simulink model "power_wind_dfig"  (R2016a)
settings: Solver=ode23tb  StartTime=0.0  StopTime=100  FixedStep=1/60  MaxStep=1/60  RelTol=1e-4  AbsTol=1e-3
InitFcn:
  | xInitial = init_power_wind_dfig;
undefined symbols (not defined in the file): b0, D1, D11, Delta, F, find_system, Fnom, gcbh, H, ILd_init, ILq_init, Imax_grid_conv, Init, j, Kd, Ki_dc_reg, Ki_grid_side_cur_reg, Ki_power_reg, Ki_Q, Ki_rotor_side_cur_reg, Ki_volt_reg, Kp, Kp_dc_reg, Kp_grid_side_cur_reg, Kp_power_reg, Kp_Q, Kp_rotor_side_cur_reg, Kp_volt_reg, L_RL, Llr, Lls, p, Pnom, power_A, power_B, power_D, R_RL, Rr, Rs, speed_A, speed_B, speed_C, speed_D, sps_rtmsupport, Vcontrol, Vnom, Wind_On, wo
libraries: powerlib_meascontrol x29, powerlib x27, simulink_extras x5, re_lib x2
(part 5 of 5)

== system power_wind_dfig/Plant 2 MVA/Plant & Motor Protection/AC Voltage Protection/Voltage Measurement/magnitude2/Fourier1 ==
  signal : Inport
  Constant : Constant  Value=0
  Fcn : Fcn  Expr=u^2
  Fcn1 : Fcn  Expr=u^2
  Fcn2 : Fcn  Expr=sqrt(u)
  Fcn3 : Fcn  Expr=180/pi*atan2(u[2],u[1])
  Gain1 : Gain  Gain=k*f1  SaturateOnIntegerOverflow=on  OutDataTypeStr=Inherit: Same as input  ParamDataTypeStr=Inherit: Same as input
  Integ2 : Integrator  InitialConditionSource=external
  Mux : Mux  Inputs=2
  Product : Product  SaturateOnIntegerOverflow=on  InputSameDT=on  OutDataTypeStr=Inherit: Same as first input
  Product1 : Product  SaturateOnIntegerOverflow=on  InputSameDT=on  OutDataTypeStr=Inherit: Same as first input
  Sum : Sum  SaturateOnIntegerOverflow=on  InputSameDT=on  OutDataTypeStr=Inherit: Same as first input
  Sum1 : Sum  Inputs=+-  SaturateOnIntegerOverflow=on  InputSameDT=on  OutDataTypeStr=Inherit: Same as first input
  Sum2 : Sum  Inputs=+-  SaturateOnIntegerOverflow=on  InputSameDT=on  OutDataTypeStr=Inherit: Same as first input
  T : TransportDelay  DelayTime=1/f1  BufferSize=2048
  T1 : TransportDelay  DelayTime=1/f1  BufferSize=2048
  cos(nwt) : Sin  Frequency=2*pi*n*f1  Phase=pi/2  SampleTime=0
  integ1 : Integrator  InitialConditionSource=external
  sin(nwt) : Sin  Frequency=2*pi*n*f1  SampleTime=0
  magnitude : Outport  InitialOutput=0
  angle : Outport  Port=2  InitialOutput=0
  wires:
  Constant/1 -> integ1/2, Integ2/2
  Sum/1 -> Fcn2/1
  Fcn/1 -> Sum/1
  Fcn1/1 -> Sum/2
  Mux/1 -> Fcn3/1
  Fcn3/1 -> angle/1
  sin(nwt)/1 -> Product/1
  cos(nwt)/1 -> Product1/2
  Product/1 -> integ1/1
  Product1/1 -> Integ2/1
  T/1 -> Sum1/2
  T1/1 -> Sum2/2
  integ1/1 -> Sum1/1, T/1
  Integ2/1 -> T1/1, Sum2/1
  Sum2/1 -> Fcn1/1, Mux/2
  Sum1/1 -> Fcn/1, Mux/1
  signal/1 -> Gain1/1
  Gain1/1 -> Product/2, Product1/1
  Fcn2/1 -> magnitude/1

== system power_wind_dfig/Plant 2 MVA/Plant & Motor Protection/AC Voltage Protection/Voltage Measurement/magnitude2/Fourier2 ==
  signal : Inport
  Constant : Constant  Value=0
  Fcn : Fcn  Expr=u^2
  Fcn1 : Fcn  Expr=u^2
  Fcn2 : Fcn  Expr=sqrt(u)
  Fcn3 : Fcn  Expr=180/pi*atan2(u[2],u[1])
  Gain1 : Gain  Gain=k*f1  SaturateOnIntegerOverflow=on  OutDataTypeStr=Inherit: Same as input  ParamDataTypeStr=Inherit: Same as input
  Integ2 : Integrator  InitialConditionSource=external
  Mux : Mux  Inputs=2
  Product : Product  SaturateOnIntegerOverflow=on  InputSameDT=on  OutDataTypeStr=Inherit: Same as first input
  Product1 : Product  SaturateOnIntegerOverflow=on  InputSameDT=on  OutDataTypeStr=Inherit: Same as first input
  Sum : Sum  SaturateOnIntegerOverflow=on  InputSameDT=on  OutDataTypeStr=Inherit: Same as first input
  Sum1 : Sum  Inputs=+-  SaturateOnIntegerOverflow=on  InputSameDT=on  OutDataTypeStr=Inherit: Same as first input
  Sum2 : Sum  Inputs=+-  SaturateOnIntegerOverflow=on  InputSameDT=on  OutDataTypeStr=Inherit: Same as first input
  T : TransportDelay  DelayTime=1/f1  BufferSize=2048
  T1 : TransportDelay  DelayTime=1/f1  BufferSize=2048
  cos(nwt) : Sin  Frequency=2*pi*n*f1  Phase=pi/2  SampleTime=0
  integ1 : Integrator  InitialConditionSource=external
  sin(nwt) : Sin  Frequency=2*pi*n*f1  SampleTime=0
  magnitude : Outport  InitialOutput=0
  angle : Outport  Port=2  InitialOutput=0
  wires:
  Fcn2/1 -> magnitude/1
  Gain1/1 -> Product1/1, Product/2
  signal/1 -> Gain1/1
  Sum1/1 -> Mux/1, Fcn/1
  Sum2/1 -> Mux/2, Fcn1/1
  Integ2/1 -> Sum2/1, T1/1
  integ1/1 -> T/1, Sum1/1
  T1/1 -> Sum2/2
  T/1 -> Sum1/2
  Product1/1 -> Integ2/1
  Product/1 -> integ1/1
  cos(nwt)/1 -> Product1/2
  sin(nwt)/1 -> Product/1
  Fcn3/1 -> angle/1
  Mux/1 -> Fcn3/1
  Fcn1/1 -> Sum/2
  Fcn/1 -> Sum/1
  Sum/1 -> Fcn2/1
  Constant/1 -> Integ2/2, integ1/2

== system power_wind_dfig/Wind Turbine Doubly-Fed Induction Generator (Phasor Type)1/Generator & Converters/Control/wind_dfig_grid/Current regulator/Subsystem3 ==
  In1 : Inport
  Gain : Gain  Gain=Ki  SaturateOnIntegerOverflow=on  OutDataTypeStr=Inherit: Same as input  ParamDataTypeStr=Inherit: Same as input
  Gain1 : Gain  Gain=Kp  SaturateOnIntegerOverflow=on  OutDataTypeStr=Inherit: Same as input  ParamDataTypeStr=Inherit: Same as input
  Integrator : Integrator  InitialCondition=Init  LimitOutput=on  UpperSaturationLimit=Upper_Limit  LowerSaturationLimit=Lower_Limit
  Saturation : Saturate  UpperLimit=Upper_Limit  LowerLimit=Lower_Limit
  Sum7 : Sum  SaturateOnIntegerOverflow=on  InputSameDT=on  OutDataTypeStr=Inherit: Same as first input
  Out1 : Outport
  wires:
  Saturation/1 -> Out1/1
  Sum7/1 -> Saturation/1
  In1/1 -> Gain/1, Gain1/1
  Integrator/1 -> Sum7/2
  Gain1/1 -> Sum7/1
  Gain/1 -> Integrator/1

== system power_wind_dfig/Wind Turbine Doubly-Fed Induction Generator (Phasor Type)1/Generator & Converters/Control/wind_dfig_grid/DC bus voltage Regulator/Subsystem1 ==
  In1 : Inport
  Gain : Gain  Gain=Ki  SaturateOnIntegerOverflow=on  OutDataTypeStr=Inherit: Same as input  ParamDataTypeStr=Inherit: Same as input
  Gain1 : Gain  Gain=Kp  SaturateOnIntegerOverflow=on  OutDataTypeStr=Inherit: Same as input  ParamDataTypeStr=Inherit: Same as input
  Integrator : Integrator  InitialCondition=Init  LimitOutput=on  UpperSaturationLimit=Upper_Limit  LowerSaturationLimit=Lower_Limit
  Saturation : Saturate  UpperLimit=Upper_Limit  LowerLimit=Lower_Limit
  Sum7 : Sum  SaturateOnIntegerOverflow=on  InputSameDT=on  OutDataTypeStr=Inherit: Same as first input
  Out1 : Outport
  wires:
  Saturation/1 -> Out1/1
  Sum7/1 -> Saturation/1
  In1/1 -> Gain/1, Gain1/1
  Integrator/1 -> Sum7/2
  Gain1/1 -> Sum7/1
  Gain/1 -> Integrator/1

== system power_wind_dfig/Wind Turbine Doubly-Fed Induction Generator (Phasor Type)1/Generator & Converters/Control/wind_dfig_rotor/Current Regulator/Subsystem1 ==
  In1 : Inport
  Gain : Gain  Gain=Ki  SaturateOnIntegerOverflow=on  OutDataTypeStr=Inherit: Same as input  ParamDataTypeStr=Inherit: Same as input
  Gain1 : Gain  Gain=Kp  SaturateOnIntegerOverflow=on  OutDataTypeStr=Inherit: Same as input  ParamDataTypeStr=Inherit: Same as input
  Integrator : Integrator  InitialCondition=Init  LimitOutput=on  UpperSaturationLimit=Upper_Limit  LowerSaturationLimit=Lower_Limit
  Saturation : Saturate  UpperLimit=Upper_Limit  LowerLimit=Lower_Limit
  Sum7 : Sum  SaturateOnIntegerOverflow=on  InputSameDT=on  OutDataTypeStr=Inherit: Same as first input
  Out1 : Outport
  wires:
  Saturation/1 -> Out1/1
  Sum7/1 -> Saturation/1
  In1/1 -> Gain/1, Gain1/1
  Integrator/1 -> Sum7/2
  Gain1/1 -> Sum7/1
  Gain/1 -> Integrator/1

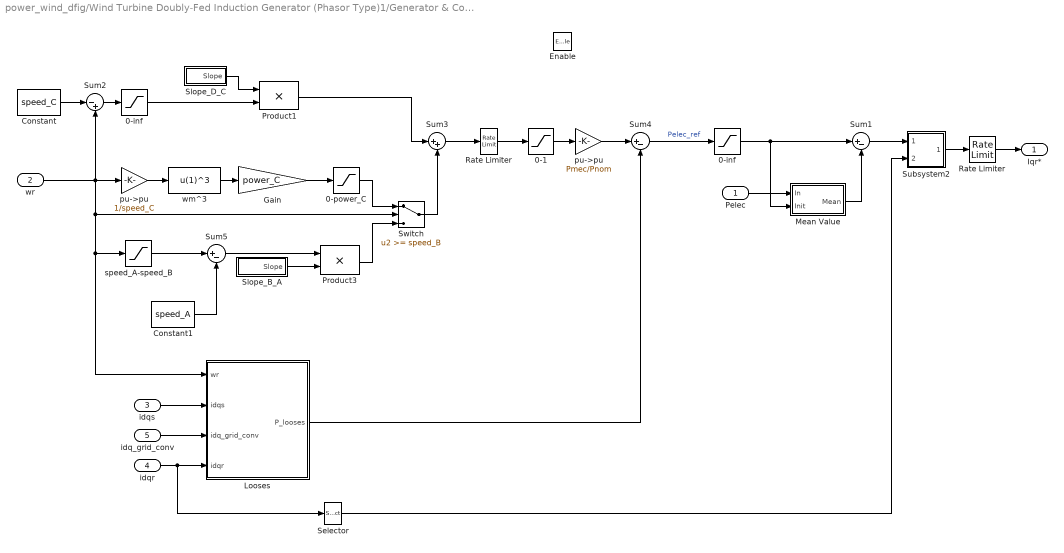
== system power_wind_dfig/Wind Turbine Doubly-Fed Induction Generator (Phasor Type)1/Generator & Converters/Control/wind_dfig_rotor/Power Regulator/Subsystem ==
  Pelec : Inport
  wr : Inport  Port=2
  idqs : Inport  Port=3
  idqr : Inport  Port=4
  idq_grid_conv : Inport  Port=5
  Enable : EnablePort  PropagateVarSize=During execution
  0-1 : Saturate  UpperLimit=1  LowerLimit=0
  0-inf : Saturate  UpperLimit=inf  LowerLimit=0
  "0-inf " : Saturate  UpperLimit=inf  LowerLimit=0
  0-power_C : Saturate  UpperLimit=power_C  LowerLimit=0
  Constant : Constant  Value=speed_C
  Constant1 : Constant  Value=speed_A
  "Gain " : Gain  Gain=power_C  SaturateOnIntegerOverflow=on  OutDataTypeStr=Inherit: Same as input  ParamDataTypeStr=Inherit: Same as input
  Looses : Subsystem
  Mean Value : Subsystem  mask(Mean value){Period=1/Fnom}
      mask prompts: Period "Averaging period (s):"
      mask help: This block uses the running window averaging technique to compute the mean value of the input signal over the specified period.
  Product1 : Product  SaturateOnIntegerOverflow=on  OutDataTypeStr=Inherit: Same as first input
  Product3 : Product  SaturateOnIntegerOverflow=on  OutDataTypeStr=Inherit: Same as first input
  Rate Limiter : RateLimiter  RisingSlewLimit=current_slew_rate  FallingSlewLimit=-current_slew_rate
  "Rate Limiter " : RateLimiter  RisingSlewLimit=power_slew_rate  FallingSlewLimit=-power_slew_rate
  Selector : Selector  InputPortWidth=2  IndexOptions=Index vector (dialog)  Indices=2  OutputSizes=1
  Slope_B_A : Subsystem
  Slope_D_C : Subsystem
  Subsystem2 : Subsystem  mask{Kp=Kp_power_reg, Ki=Ki_power_reg, Limits=[1 0]}
      mask prompts: Kp "Proportional gain (Kp):"; Ki "Integral gain (Ki):"; Limits "Output limits [Upper Lower]:"
      mask init:
      | Upper_Limit=Limits(1);
      | Lower_Limit=Limits(2);
      mask Display: disp('PI')
  Sum1 : Sum  Inputs=|+-  SaturateOnIntegerOverflow=on
  Sum2 : Sum  Inputs=|-+  SaturateOnIntegerOverflow=on
  Sum3 : Sum  Inputs=|++  SaturateOnIntegerOverflow=on
  Sum4 : Sum  Inputs=|+-  SaturateOnIntegerOverflow=on
  Sum5 : Sum  Inputs=|+-  SaturateOnIntegerOverflow=on
  Switch : Switch  Threshold=speed_B  SaturateOnIntegerOverflow=on
  "pu->pu " : Gain  Gain=1/speed_C  SaturateOnIntegerOverflow=on  OutDataTypeStr=Inherit: Same as input  ParamDataTypeStr=Inherit: Same as input
  "pu->pu  " : Gain  Gain=Pmec/Pnom  SaturateOnIntegerOverflow=on  OutDataTypeStr=Inherit: Same as input  ParamDataTypeStr=Inherit: Same as input
  speed_A-speed_B : Saturate  UpperLimit=speed_B  LowerLimit=speed_A
  wm^3 : Fcn  Expr=u(1)^3
  Iqr* : Outport
  wires:
  Product1/1 -> Sum3/1
  0-inf/1 -> Product1/2
  Sum2/1 -> 0-inf/1
  Constant/1 -> Sum2/1
  "Gain "/1 -> 0-power_C/1
  Mean Value/1(Mean) -> Sum1/2
  Selector/1 -> Subsystem2/2(Init)
  Subsystem2/1(Out1) -> Rate Limiter/1
  Sum1/1 -> Subsystem2/1(In1)
  Looses/1(P_looses) -> Sum4/2
  Pelec/1 -> Mean Value/1(In)
  idq_grid_conv/1 -> Looses/3(idq_grid_conv)
  idqr/1 -> Selector/1, Looses/4(idqr)
  idqs/1 -> Looses/2(idqs)
  Sum4/1 -> "0-inf "/1  "Pelec_ref"
  wm^3/1 -> "Gain "/1
  "pu->pu "/1 -> wm^3/1
  Rate Limiter/1 -> Iqr*/1
  Sum3/1 -> "Rate Limiter "/1
  "pu->pu  "/1 -> Sum4/1
  "Rate Limiter "/1 -> 0-1/1
  0-1/1 -> "pu->pu  "/1
  wr/1 -> "pu->pu "/1, Sum2/2, speed_A-speed_B/1, Looses/1(wr), Switch/2
  0-power_C/1 -> Switch/1
  Product3/1 -> Switch/3
  Constant1/1 -> Sum5/2
  speed_A-speed_B/1 -> Sum5/1
  Sum5/1 -> Product3/1
  Switch/1 -> Sum3/2
  Slope_D_C/1(Slope) -> Product1/1
  Slope_B_A/1(Slope) -> Product3/2
  "0-inf "/1 -> Mean Value/2(Init), Sum1/1

== system power_wind_dfig/Wind Turbine Doubly-Fed Induction Generator (Phasor Type)1/Generator & Converters/Control/wind_dfig_rotor/Power Regulator/Subsystem  ==
  Pelec : Inport
  idqr : Inport  Port=2
  Power_opt : Inport  Port=3
  Enable : EnablePort  PropagateVarSize=During execution
  Mean Value : Subsystem  mask(Mean value){Period=1/Fnom}
      mask prompts: Period "Averaging period (s):"
      mask help: This block uses the running window averaging technique to compute the mean value of the input signal over the specified period.
  Rate Limiter : RateLimiter  RisingSlewLimit=current_slew_rate  FallingSlewLimit=-current_slew_rate
  Selector : Selector  InputPortWidth=2  IndexOptions=Index vector (dialog)  Indices=2  OutputSizes=1
  Subsystem2 : Subsystem  mask{Kp=Kp_power_reg, Ki=Ki_power_reg, Limits=[1 0]}
      mask prompts: Kp "Proportional gain (Kp):"; Ki "Integral gain (Ki):"; Limits "Output limits [Upper Lower]:"
      mask init:
      | Upper_Limit=Limits(1);
      | Lower_Limit=Limits(2);
      mask Display: disp('PI')
  Sum1 : Sum  Inputs=|+-  SaturateOnIntegerOverflow=on
  Iqr* : Outport
  wires:
  Mean Value/1(Mean) -> Sum1/2
  idqr/1 -> Selector/1
  Subsystem2/1(Out1) -> Rate Limiter/1
  Power_opt/1 -> Mean Value/2(Init), Sum1/1
  Selector/1 -> Subsystem2/2(Init)
  Pelec/1 -> Mean Value/1(In)
  Sum1/1 -> Subsystem2/1(In1)
  Rate Limiter/1 -> Iqr*/1

== system power_wind_dfig/Wind Turbine Doubly-Fed Induction Generator (Phasor Type)1/Generator & Converters/Control/wind_dfig_rotor/Q Regulator/Mean Value ==
  note: Mean value
  In : Inport
  Init : Inport  Port=2
  Gain : Gain  Gain=1/Period  SaturateOnIntegerOverflow=on  OutDataTypeStr=Inherit: Same as input  ParamDataTypeStr=Inherit: Same as input
  Step : Step  Time=Period+eps  SampleTime=0
  Sum : Sum  Inputs=+-  SaturateOnIntegerOverflow=on  InputSameDT=on  OutDataTypeStr=Inherit: Same as first input
  Switch : Switch  Threshold=0.5  SaturateOnIntegerOverflow=on
  Transport Delay : TransportDelay  DelayTime=Period
  integrator : Integrator
  Mean : Outport
  wires:
  Transport Delay/1 -> Sum/2
  integrator/1 -> Transport Delay/1, Sum/1
  In/1 -> integrator/1
  Sum/1 -> Gain/1
  Gain/1 -> Switch/1
  Switch/1 -> Mean/1
  Step/1 -> Switch/2
  Init/1 -> Switch/3

== system power_wind_dfig/Wind Turbine Doubly-Fed Induction Generator (Phasor Type)1/Generator & Converters/Control/wind_dfig_rotor/Q Regulator/Subsystem1 ==
  In1 : Inport
  Init : Inport  Port=2
  Gain : Gain  Gain=Ki  SaturateOnIntegerOverflow=on  OutDataTypeStr=Inherit: Same as input  ParamDataTypeStr=Inherit: Same as input
  Gain1 : Gain  Gain=Kp  SaturateOnIntegerOverflow=on  OutDataTypeStr=Inherit: Same as input  ParamDataTypeStr=Inherit: Same as input
  Integrator : Integrator  InitialConditionSource=external  InitialCondition=Init  LimitOutput=on  UpperSaturationLimit=Upper_Limit  LowerSaturationLimit=Lower_Limit
  Saturation : Saturate  UpperLimit=Upper_Limit  LowerLimit=Lower_Limit
  Sum7 : Sum  SaturateOnIntegerOverflow=on  InputSameDT=on  OutDataTypeStr=Inherit: Same as first input
  Out1 : Outport
  wires:
  Init/1 -> Integrator/2
  Saturation/1 -> Out1/1
  Sum7/1 -> Saturation/1
  In1/1 -> Gain/1, Gain1/1
  Integrator/1 -> Sum7/2
  Gain1/1 -> Sum7/1
  Gain/1 -> Integrator/1

== system power_wind_dfig/Wind Turbine Doubly-Fed Induction Generator (Phasor Type)1/Generator & Converters/Control/wind_dfig_rotor/V Regulator/Mean Value ==
  note: Mean value
  In : Inport
  Init : Inport  Port=2
  Gain : Gain  Gain=1/Period  SaturateOnIntegerOverflow=on  OutDataTypeStr=Inherit: Same as input  ParamDataTypeStr=Inherit: Same as input
  Step : Step  Time=Period+eps  SampleTime=0
  Sum : Sum  Inputs=+-  SaturateOnIntegerOverflow=on  InputSameDT=on  OutDataTypeStr=Inherit: Same as first input
  Switch : Switch  Threshold=0.5  SaturateOnIntegerOverflow=on
  Transport Delay : TransportDelay  DelayTime=Period
  integrator : Integrator
  Mean : Outport
  wires:
  Transport Delay/1 -> Sum/2
  integrator/1 -> Transport Delay/1, Sum/1
  In/1 -> integrator/1
  Sum/1 -> Gain/1
  Gain/1 -> Switch/1
  Switch/1 -> Mean/1
  Step/1 -> Switch/2
  Init/1 -> Switch/3

== system power_wind_dfig/Wind Turbine Doubly-Fed Induction Generator (Phasor Type)1/Generator & Converters/Control/wind_dfig_rotor/V Regulator/Mean Value1 ==
  note: Mean value
  In : Inport
  Init : Inport  Port=2
  Gain : Gain  Gain=1/Period  SaturateOnIntegerOverflow=on  OutDataTypeStr=Inherit: Same as input  ParamDataTypeStr=Inherit: Same as input
  Step : Step  Time=Period+eps  SampleTime=0
  Sum : Sum  Inputs=+-  SaturateOnIntegerOverflow=on  InputSameDT=on  OutDataTypeStr=Inherit: Same as first input
  Switch : Switch  Threshold=0.5  SaturateOnIntegerOverflow=on
  Transport Delay : TransportDelay  DelayTime=Period
  integrator : Integrator
  Mean : Outport
  wires:
  Init/1 -> Switch/3
  Step/1 -> Switch/2
  Switch/1 -> Mean/1
  Gain/1 -> Switch/1
  Sum/1 -> Gain/1
  In/1 -> integrator/1
  integrator/1 -> Sum/1, Transport Delay/1
  Transport Delay/1 -> Sum/2

== system power_wind_dfig/Wind Turbine Doubly-Fed Induction Generator (Phasor Type)1/Generator & Converters/Control/wind_dfig_rotor/V Regulator/Subsystem1 ==
  In1 : Inport
  Init : Inport  Port=2
  Gain : Gain  Gain=Ki  SaturateOnIntegerOverflow=on  OutDataTypeStr=Inherit: Same as input  ParamDataTypeStr=Inherit: Same as input
  Gain1 : Gain  Gain=Kp  SaturateOnIntegerOverflow=on  OutDataTypeStr=Inherit: Same as input  ParamDataTypeStr=Inherit: Same as input
  Integrator : Integrator  InitialConditionSource=external  InitialCondition=Init  LimitOutput=on  UpperSaturationLimit=Upper_Limit  LowerSaturationLimit=Lower_Limit
  Saturation : Saturate  UpperLimit=Upper_Limit  LowerLimit=Lower_Limit
  Sum7 : Sum  SaturateOnIntegerOverflow=on  InputSameDT=on  OutDataTypeStr=Inherit: Same as first input
  Out1 : Outport
  wires:
  Gain/1 -> Integrator/1
  Gain1/1 -> Sum7/1
  Integrator/1 -> Sum7/2
  In1/1 -> Gain1/1, Gain/1
  Sum7/1 -> Saturation/1
  Saturation/1 -> Out1/1
  Init/1 -> Integrator/2

== system power_wind_dfig/Wind Turbine Protection/Protection System/AC Current Protection/Current Measurement/magnitude/Fourier1 ==
  signal : Inport
  Constant : Constant  Value=0
  Fcn : Fcn  Expr=u^2
  Fcn1 : Fcn  Expr=u^2
  Fcn2 : Fcn  Expr=sqrt(u)
  Fcn3 : Fcn  Expr=180/pi*atan2(u[2],u[1])
  Gain1 : Gain  Gain=k*f1  SaturateOnIntegerOverflow=on  OutDataTypeStr=Inherit: Same as input  ParamDataTypeStr=Inherit: Same as input
  Integ2 : Integrator  InitialConditionSource=external
  Mux : Mux  Inputs=2
  Product : Product  SaturateOnIntegerOverflow=on  InputSameDT=on  OutDataTypeStr=Inherit: Same as first input
  Product1 : Product  SaturateOnIntegerOverflow=on  InputSameDT=on  OutDataTypeStr=Inherit: Same as first input
  Sum : Sum  SaturateOnIntegerOverflow=on  InputSameDT=on  OutDataTypeStr=Inherit: Same as first input
  Sum1 : Sum  Inputs=+-  SaturateOnIntegerOverflow=on  InputSameDT=on  OutDataTypeStr=Inherit: Same as first input
  Sum2 : Sum  Inputs=+-  SaturateOnIntegerOverflow=on  InputSameDT=on  OutDataTypeStr=Inherit: Same as first input
  T : TransportDelay  DelayTime=1/f1  BufferSize=2048
  T1 : TransportDelay  DelayTime=1/f1  BufferSize=2048
  cos(nwt) : Sin  Frequency=2*pi*n*f1  Phase=pi/2  SampleTime=0
  integ1 : Integrator  InitialConditionSource=external
  sin(nwt) : Sin  Frequency=2*pi*n*f1  SampleTime=0
  magnitude : Outport  InitialOutput=0
  angle : Outport  Port=2  InitialOutput=0
  wires:
  Fcn2/1 -> magnitude/1
  Gain1/1 -> Product1/1, Product/2
  signal/1 -> Gain1/1
  Sum1/1 -> Mux/1, Fcn/1
  Sum2/1 -> Mux/2, Fcn1/1
  Integ2/1 -> Sum2/1, T1/1
  integ1/1 -> T/1, Sum1/1
  T1/1 -> Sum2/2
  T/1 -> Sum1/2
  Product1/1 -> Integ2/1
  Product/1 -> integ1/1
  cos(nwt)/1 -> Product1/2
  sin(nwt)/1 -> Product/1
  Fcn3/1 -> angle/1
  Mux/1 -> Fcn3/1
  Fcn1/1 -> Sum/2
  Fcn/1 -> Sum/1
  Sum/1 -> Fcn2/1
  Constant/1 -> Integ2/2, integ1/2

== system power_wind_dfig/Wind Turbine Protection/Protection System/AC Current Protection/Current Measurement/magnitude/Fourier2 ==
  signal : Inport
  Constant : Constant  Value=0
  Fcn : Fcn  Expr=u^2
  Fcn1 : Fcn  Expr=u^2
  Fcn2 : Fcn  Expr=sqrt(u)
  Fcn3 : Fcn  Expr=180/pi*atan2(u[2],u[1])
  Gain1 : Gain  Gain=k*f1  SaturateOnIntegerOverflow=on  OutDataTypeStr=Inherit: Same as input  ParamDataTypeStr=Inherit: Same as input
  Integ2 : Integrator  InitialConditionSource=external
  Mux : Mux  Inputs=2
  Product : Product  SaturateOnIntegerOverflow=on  InputSameDT=on  OutDataTypeStr=Inherit: Same as first input
  Product1 : Product  SaturateOnIntegerOverflow=on  InputSameDT=on  OutDataTypeStr=Inherit: Same as first input
  Sum : Sum  SaturateOnIntegerOverflow=on  InputSameDT=on  OutDataTypeStr=Inherit: Same as first input
  Sum1 : Sum  Inputs=+-  SaturateOnIntegerOverflow=on  InputSameDT=on  OutDataTypeStr=Inherit: Same as first input
  Sum2 : Sum  Inputs=+-  SaturateOnIntegerOverflow=on  InputSameDT=on  OutDataTypeStr=Inherit: Same as first input
  T : TransportDelay  DelayTime=1/f1  BufferSize=2048
  T1 : TransportDelay  DelayTime=1/f1  BufferSize=2048
  cos(nwt) : Sin  Frequency=2*pi*n*f1  Phase=pi/2  SampleTime=0
  integ1 : Integrator  InitialConditionSource=external
  sin(nwt) : Sin  Frequency=2*pi*n*f1  SampleTime=0
  magnitude : Outport  InitialOutput=0
  angle : Outport  Port=2  InitialOutput=0
  wires:
  Constant/1 -> integ1/2, Integ2/2
  Sum/1 -> Fcn2/1
  Fcn/1 -> Sum/1
  Fcn1/1 -> Sum/2
  Mux/1 -> Fcn3/1
  Fcn3/1 -> angle/1
  sin(nwt)/1 -> Product/1
  cos(nwt)/1 -> Product1/2
  Product/1 -> integ1/1
  Product1/1 -> Integ2/1
  T/1 -> Sum1/2
  T1/1 -> Sum2/2
  integ1/1 -> Sum1/1, T/1
  Integ2/1 -> T1/1, Sum2/1
  Sum2/1 -> Fcn1/1, Mux/2
  Sum1/1 -> Fcn/1, Mux/1
  signal/1 -> Gain1/1
  Gain1/1 -> Product/2, Product1/1
  Fcn2/1 -> magnitude/1

== system power_wind_dfig/Wind Turbine Protection/Protection System/AC Current Protection/Current Measurement/magnitude1/Fourier1 ==
  signal : Inport
  Constant : Constant  Value=0
  Fcn : Fcn  Expr=u^2
  Fcn1 : Fcn  Expr=u^2
  Fcn2 : Fcn  Expr=sqrt(u)
  Fcn3 : Fcn  Expr=180/pi*atan2(u[2],u[1])
  Gain1 : Gain  Gain=k*f1  SaturateOnIntegerOverflow=on  OutDataTypeStr=Inherit: Same as input  ParamDataTypeStr=Inherit: Same as input
  Integ2 : Integrator  InitialConditionSource=external
  Mux : Mux  Inputs=2
  Product : Product  SaturateOnIntegerOverflow=on  InputSameDT=on  OutDataTypeStr=Inherit: Same as first input
  Product1 : Product  SaturateOnIntegerOverflow=on  InputSameDT=on  OutDataTypeStr=Inherit: Same as first input
  Sum : Sum  SaturateOnIntegerOverflow=on  InputSameDT=on  OutDataTypeStr=Inherit: Same as first input
  Sum1 : Sum  Inputs=+-  SaturateOnIntegerOverflow=on  InputSameDT=on  OutDataTypeStr=Inherit: Same as first input
  Sum2 : Sum  Inputs=+-  SaturateOnIntegerOverflow=on  InputSameDT=on  OutDataTypeStr=Inherit: Same as first input
  T : TransportDelay  DelayTime=1/f1  BufferSize=2048
  T1 : TransportDelay  DelayTime=1/f1  BufferSize=2048
  cos(nwt) : Sin  Frequency=2*pi*n*f1  Phase=pi/2  SampleTime=0
  integ1 : Integrator  InitialConditionSource=external
  sin(nwt) : Sin  Frequency=2*pi*n*f1  SampleTime=0
  magnitude : Outport  InitialOutput=0
  angle : Outport  Port=2  InitialOutput=0
  wires:
  Constant/1 -> integ1/2, Integ2/2
  Sum/1 -> Fcn2/1
  Fcn/1 -> Sum/1
  Fcn1/1 -> Sum/2
  Mux/1 -> Fcn3/1
  Fcn3/1 -> angle/1
  sin(nwt)/1 -> Product/1
  cos(nwt)/1 -> Product1/2
  Product/1 -> integ1/1
  Product1/1 -> Integ2/1
  T/1 -> Sum1/2
  T1/1 -> Sum2/2
  integ1/1 -> Sum1/1, T/1
  Integ2/1 -> T1/1, Sum2/1
  Sum2/1 -> Fcn1/1, Mux/2
  Sum1/1 -> Fcn/1, Mux/1
  signal/1 -> Gain1/1
  Gain1/1 -> Product/2, Product1/1
  Fcn2/1 -> magnitude/1

== system power_wind_dfig/Wind Turbine Protection/Protection System/AC Current Protection/Current Measurement/magnitude1/Fourier2 ==
  signal : Inport
  Constant : Constant  Value=0
  Fcn : Fcn  Expr=u^2
  Fcn1 : Fcn  Expr=u^2
  Fcn2 : Fcn  Expr=sqrt(u)
  Fcn3 : Fcn  Expr=180/pi*atan2(u[2],u[1])
  Gain1 : Gain  Gain=k*f1  SaturateOnIntegerOverflow=on  OutDataTypeStr=Inherit: Same as input  ParamDataTypeStr=Inherit: Same as input
  Integ2 : Integrator  InitialConditionSource=external
  Mux : Mux  Inputs=2
  Product : Product  SaturateOnIntegerOverflow=on  InputSameDT=on  OutDataTypeStr=Inherit: Same as first input
  Product1 : Product  SaturateOnIntegerOverflow=on  InputSameDT=on  OutDataTypeStr=Inherit: Same as first input
  Sum : Sum  SaturateOnIntegerOverflow=on  InputSameDT=on  OutDataTypeStr=Inherit: Same as first input
  Sum1 : Sum  Inputs=+-  SaturateOnIntegerOverflow=on  InputSameDT=on  OutDataTypeStr=Inherit: Same as first input
  Sum2 : Sum  Inputs=+-  SaturateOnIntegerOverflow=on  InputSameDT=on  OutDataTypeStr=Inherit: Same as first input
  T : TransportDelay  DelayTime=1/f1  BufferSize=2048
  T1 : TransportDelay  DelayTime=1/f1  BufferSize=2048
  cos(nwt) : Sin  Frequency=2*pi*n*f1  Phase=pi/2  SampleTime=0
  integ1 : Integrator  InitialConditionSource=external
  sin(nwt) : Sin  Frequency=2*pi*n*f1  SampleTime=0
  magnitude : Outport  InitialOutput=0
  angle : Outport  Port=2  InitialOutput=0
  wires:
  Fcn2/1 -> magnitude/1
  Gain1/1 -> Product1/1, Product/2
  signal/1 -> Gain1/1
  Sum1/1 -> Mux/1, Fcn/1
  Sum2/1 -> Mux/2, Fcn1/1
  Integ2/1 -> Sum2/1, T1/1
  integ1/1 -> T/1, Sum1/1
  T1/1 -> Sum2/2
  T/1 -> Sum1/2
  Product1/1 -> Integ2/1
  Product/1 -> integ1/1
  cos(nwt)/1 -> Product1/2
  sin(nwt)/1 -> Product/1
  Fcn3/1 -> angle/1
  Mux/1 -> Fcn3/1
  Fcn1/1 -> Sum/2
  Fcn/1 -> Sum/1
  Sum/1 -> Fcn2/1
  Constant/1 -> Integ2/2, integ1/2

== system power_wind_dfig/Wind Turbine Protection/Protection System/AC Voltage Protection/Voltage Measurement/magnitude/Fourier1 ==
  signal : Inport
  Constant : Constant  Value=0
  Fcn : Fcn  Expr=u^2
  Fcn1 : Fcn  Expr=u^2
  Fcn2 : Fcn  Expr=sqrt(u)
  Fcn3 : Fcn  Expr=180/pi*atan2(u[2],u[1])
  Gain1 : Gain  Gain=k*f1  SaturateOnIntegerOverflow=on  OutDataTypeStr=Inherit: Same as input  ParamDataTypeStr=Inherit: Same as input
  Integ2 : Integrator  InitialConditionSource=external
  Mux : Mux  Inputs=2
  Product : Product  SaturateOnIntegerOverflow=on  InputSameDT=on  OutDataTypeStr=Inherit: Same as first input
  Product1 : Product  SaturateOnIntegerOverflow=on  InputSameDT=on  OutDataTypeStr=Inherit: Same as first input
  Sum : Sum  SaturateOnIntegerOverflow=on  InputSameDT=on  OutDataTypeStr=Inherit: Same as first input
  Sum1 : Sum  Inputs=+-  SaturateOnIntegerOverflow=on  InputSameDT=on  OutDataTypeStr=Inherit: Same as first input
  Sum2 : Sum  Inputs=+-  SaturateOnIntegerOverflow=on  InputSameDT=on  OutDataTypeStr=Inherit: Same as first input
  T : TransportDelay  DelayTime=1/f1  BufferSize=2048
  T1 : TransportDelay  DelayTime=1/f1  BufferSize=2048
  cos(nwt) : Sin  Frequency=2*pi*n*f1  Phase=pi/2  SampleTime=0
  integ1 : Integrator  InitialConditionSource=external
  sin(nwt) : Sin  Frequency=2*pi*n*f1  SampleTime=0
  magnitude : Outport  InitialOutput=0
  angle : Outport  Port=2  InitialOutput=0
  wires:
  Fcn2/1 -> magnitude/1
  Gain1/1 -> Product1/1, Product/2
  signal/1 -> Gain1/1
  Sum1/1 -> Mux/1, Fcn/1
  Sum2/1 -> Mux/2, Fcn1/1
  Integ2/1 -> Sum2/1, T1/1
  integ1/1 -> T/1, Sum1/1
  T1/1 -> Sum2/2
  T/1 -> Sum1/2
  Product1/1 -> Integ2/1
  Product/1 -> integ1/1
  cos(nwt)/1 -> Product1/2
  sin(nwt)/1 -> Product/1
  Fcn3/1 -> angle/1
  Mux/1 -> Fcn3/1
  Fcn1/1 -> Sum/2
  Fcn/1 -> Sum/1
  Sum/1 -> Fcn2/1
  Constant/1 -> Integ2/2, integ1/2

== system power_wind_dfig/Wind Turbine Protection/Protection System/AC Voltage Protection/Voltage Measurement/magnitude/Fourier2 ==
  signal : Inport
  Constant : Constant  Value=0
  Fcn : Fcn  Expr=u^2
  Fcn1 : Fcn  Expr=u^2
  Fcn2 : Fcn  Expr=sqrt(u)
  Fcn3 : Fcn  Expr=180/pi*atan2(u[2],u[1])
  Gain1 : Gain  Gain=k*f1  SaturateOnIntegerOverflow=on  OutDataTypeStr=Inherit: Same as input  ParamDataTypeStr=Inherit: Same as input
  Integ2 : Integrator  InitialConditionSource=external
  Mux : Mux  Inputs=2
  Product : Product  SaturateOnIntegerOverflow=on  InputSameDT=on  OutDataTypeStr=Inherit: Same as first input
  Product1 : Product  SaturateOnIntegerOverflow=on  InputSameDT=on  OutDataTypeStr=Inherit: Same as first input
  Sum : Sum  SaturateOnIntegerOverflow=on  InputSameDT=on  OutDataTypeStr=Inherit: Same as first input
  Sum1 : Sum  Inputs=+-  SaturateOnIntegerOverflow=on  InputSameDT=on  OutDataTypeStr=Inherit: Same as first input
  Sum2 : Sum  Inputs=+-  SaturateOnIntegerOverflow=on  InputSameDT=on  OutDataTypeStr=Inherit: Same as first input
  T : TransportDelay  DelayTime=1/f1  BufferSize=2048
  T1 : TransportDelay  DelayTime=1/f1  BufferSize=2048
  cos(nwt) : Sin  Frequency=2*pi*n*f1  Phase=pi/2  SampleTime=0
  integ1 : Integrator  InitialConditionSource=external
  sin(nwt) : Sin  Frequency=2*pi*n*f1  SampleTime=0
  magnitude : Outport  InitialOutput=0
  angle : Outport  Port=2  InitialOutput=0
  wires:
  Constant/1 -> integ1/2, Integ2/2
  Sum/1 -> Fcn2/1
  Fcn/1 -> Sum/1
  Fcn1/1 -> Sum/2
  Mux/1 -> Fcn3/1
  Fcn3/1 -> angle/1
  sin(nwt)/1 -> Product/1
  cos(nwt)/1 -> Product1/2
  Product/1 -> integ1/1
  Product1/1 -> Integ2/1
  T/1 -> Sum1/2
  T1/1 -> Sum2/2
  integ1/1 -> Sum1/1, T/1
  Integ2/1 -> T1/1, Sum2/1
  Sum2/1 -> Fcn1/1, Mux/2
  Sum1/1 -> Fcn/1, Mux/1
  signal/1 -> Gain1/1
  Gain1/1 -> Product/2, Product1/1
  Fcn2/1 -> magnitude/1

== system power_wind_dfig/Wind Turbine Protection/Protection System/AC Voltage Protection/Voltage Measurement/magnitude1/Fourier1 ==
  signal : Inport
  Constant : Constant  Value=0
  Fcn : Fcn  Expr=u^2
  Fcn1 : Fcn  Expr=u^2
  Fcn2 : Fcn  Expr=sqrt(u)
  Fcn3 : Fcn  Expr=180/pi*atan2(u[2],u[1])
  Gain1 : Gain  Gain=k*f1  SaturateOnIntegerOverflow=on  OutDataTypeStr=Inherit: Same as input  ParamDataTypeStr=Inherit: Same as input
  Integ2 : Integrator  InitialConditionSource=external
  Mux : Mux  Inputs=2
  Product : Product  SaturateOnIntegerOverflow=on  InputSameDT=on  OutDataTypeStr=Inherit: Same as first input
  Product1 : Product  SaturateOnIntegerOverflow=on  InputSameDT=on  OutDataTypeStr=Inherit: Same as first input
  Sum : Sum  SaturateOnIntegerOverflow=on  InputSameDT=on  OutDataTypeStr=Inherit: Same as first input
  Sum1 : Sum  Inputs=+-  SaturateOnIntegerOverflow=on  InputSameDT=on  OutDataTypeStr=Inherit: Same as first input
  Sum2 : Sum  Inputs=+-  SaturateOnIntegerOverflow=on  InputSameDT=on  OutDataTypeStr=Inherit: Same as first input
  T : TransportDelay  DelayTime=1/f1  BufferSize=2048
  T1 : TransportDelay  DelayTime=1/f1  BufferSize=2048
  cos(nwt) : Sin  Frequency=2*pi*n*f1  Phase=pi/2  SampleTime=0
  integ1 : Integrator  InitialConditionSource=external
  sin(nwt) : Sin  Frequency=2*pi*n*f1  SampleTime=0
  magnitude : Outport  InitialOutput=0
  angle : Outport  Port=2  InitialOutput=0
  wires:
  Constant/1 -> integ1/2, Integ2/2
  Sum/1 -> Fcn2/1
  Fcn/1 -> Sum/1
  Fcn1/1 -> Sum/2
  Mux/1 -> Fcn3/1
  Fcn3/1 -> angle/1
  sin(nwt)/1 -> Product/1
  cos(nwt)/1 -> Product1/2
  Product/1 -> integ1/1
  Product1/1 -> Integ2/1
  T/1 -> Sum1/2
  T1/1 -> Sum2/2
  integ1/1 -> Sum1/1, T/1
  Integ2/1 -> T1/1, Sum2/1
  Sum2/1 -> Fcn1/1, Mux/2
  Sum1/1 -> Fcn/1, Mux/1
  signal/1 -> Gain1/1
  Gain1/1 -> Product/2, Product1/1
  Fcn2/1 -> magnitude/1

== system power_wind_dfig/Wind Turbine Protection/Protection System/AC Voltage Protection/Voltage Measurement/magnitude1/Fourier2 ==
  signal : Inport
  Constant : Constant  Value=0
  Fcn : Fcn  Expr=u^2
  Fcn1 : Fcn  Expr=u^2
  Fcn2 : Fcn  Expr=sqrt(u)
  Fcn3 : Fcn  Expr=180/pi*atan2(u[2],u[1])
  Gain1 : Gain  Gain=k*f1  SaturateOnIntegerOverflow=on  OutDataTypeStr=Inherit: Same as input  ParamDataTypeStr=Inherit: Same as input
  Integ2 : Integrator  InitialConditionSource=external
  Mux : Mux  Inputs=2
  Product : Product  SaturateOnIntegerOverflow=on  InputSameDT=on  OutDataTypeStr=Inherit: Same as first input
  Product1 : Product  SaturateOnIntegerOverflow=on  InputSameDT=on  OutDataTypeStr=Inherit: Same as first input
  Sum : Sum  SaturateOnIntegerOverflow=on  InputSameDT=on  OutDataTypeStr=Inherit: Same as first input
  Sum1 : Sum  Inputs=+-  SaturateOnIntegerOverflow=on  InputSameDT=on  OutDataTypeStr=Inherit: Same as first input
  Sum2 : Sum  Inputs=+-  SaturateOnIntegerOverflow=on  InputSameDT=on  OutDataTypeStr=Inherit: Same as first input
  T : TransportDelay  DelayTime=1/f1  BufferSize=2048
  T1 : TransportDelay  DelayTime=1/f1  BufferSize=2048
  cos(nwt) : Sin  Frequency=2*pi*n*f1  Phase=pi/2  SampleTime=0
  integ1 : Integrator  InitialConditionSource=external
  sin(nwt) : Sin  Frequency=2*pi*n*f1  SampleTime=0
  magnitude : Outport  InitialOutput=0
  angle : Outport  Port=2  InitialOutput=0
  wires:
  Fcn2/1 -> magnitude/1
  Gain1/1 -> Product1/1, Product/2
  signal/1 -> Gain1/1
  Sum1/1 -> Mux/1, Fcn/1
  Sum2/1 -> Mux/2, Fcn1/1
  Integ2/1 -> Sum2/1, T1/1
  integ1/1 -> T/1, Sum1/1
  T1/1 -> Sum2/2
  T/1 -> Sum1/2
  Product1/1 -> Integ2/1
  Product/1 -> integ1/1
  cos(nwt)/1 -> Product1/2
  sin(nwt)/1 -> Product/1
  Fcn3/1 -> angle/1
  Mux/1 -> Fcn3/1
  Fcn1/1 -> Sum/2
  Fcn/1 -> Sum/1
  Sum/1 -> Fcn2/1
  Constant/1 -> Integ2/2, integ1/2

== system power_wind_dfig/Wind Turbine Protection/Protection System/AC Voltage Protection/Voltage Measurement/magnitude2/Fourier1 ==
  signal : Inport
  Constant : Constant  Value=0
  Fcn : Fcn  Expr=u^2
  Fcn1 : Fcn  Expr=u^2
  Fcn2 : Fcn  Expr=sqrt(u)
  Fcn3 : Fcn  Expr=180/pi*atan2(u[2],u[1])
  Gain1 : Gain  Gain=k*f1  SaturateOnIntegerOverflow=on  OutDataTypeStr=Inherit: Same as input  ParamDataTypeStr=Inherit: Same as input
  Integ2 : Integrator  InitialConditionSource=external
  Mux : Mux  Inputs=2
  Product : Product  SaturateOnIntegerOverflow=on  InputSameDT=on  OutDataTypeStr=Inherit: Same as first input
  Product1 : Product  SaturateOnIntegerOverflow=on  InputSameDT=on  OutDataTypeStr=Inherit: Same as first input
  Sum : Sum  SaturateOnIntegerOverflow=on  InputSameDT=on  OutDataTypeStr=Inherit: Same as first input
  Sum1 : Sum  Inputs=+-  SaturateOnIntegerOverflow=on  InputSameDT=on  OutDataTypeStr=Inherit: Same as first input
  Sum2 : Sum  Inputs=+-  SaturateOnIntegerOverflow=on  InputSameDT=on  OutDataTypeStr=Inherit: Same as first input
  T : TransportDelay  DelayTime=1/f1  BufferSize=2048
  T1 : TransportDelay  DelayTime=1/f1  BufferSize=2048
  cos(nwt) : Sin  Frequency=2*pi*n*f1  Phase=pi/2  SampleTime=0
  integ1 : Integrator  InitialConditionSource=external
  sin(nwt) : Sin  Frequency=2*pi*n*f1  SampleTime=0
  magnitude : Outport  InitialOutput=0
  angle : Outport  Port=2  InitialOutput=0
  wires:
  Fcn2/1 -> magnitude/1
  Gain1/1 -> Product1/1, Product/2
  signal/1 -> Gain1/1
  Sum1/1 -> Mux/1, Fcn/1
  Sum2/1 -> Mux/2, Fcn1/1
  Integ2/1 -> Sum2/1, T1/1
  integ1/1 -> T/1, Sum1/1
  T1/1 -> Sum2/2
  T/1 -> Sum1/2
  Product1/1 -> Integ2/1
  Product/1 -> integ1/1
  cos(nwt)/1 -> Product1/2
  sin(nwt)/1 -> Product/1
  Fcn3/1 -> angle/1
  Mux/1 -> Fcn3/1
  Fcn1/1 -> Sum/2
  Fcn/1 -> Sum/1
  Sum/1 -> Fcn2/1
  Constant/1 -> Integ2/2, integ1/2

== system power_wind_dfig/Wind Turbine Protection/Protection System/AC Voltage Protection/Voltage Measurement/magnitude2/Fourier2 ==
  signal : Inport
  Constant : Constant  Value=0
  Fcn : Fcn  Expr=u^2
  Fcn1 : Fcn  Expr=u^2
  Fcn2 : Fcn  Expr=sqrt(u)
  Fcn3 : Fcn  Expr=180/pi*atan2(u[2],u[1])
  Gain1 : Gain  Gain=k*f1  SaturateOnIntegerOverflow=on  OutDataTypeStr=Inherit: Same as input  ParamDataTypeStr=Inherit: Same as input
  Integ2 : Integrator  InitialConditionSource=external
  Mux : Mux  Inputs=2
  Product : Product  SaturateOnIntegerOverflow=on  InputSameDT=on  OutDataTypeStr=Inherit: Same as first input
  Product1 : Product  SaturateOnIntegerOverflow=on  InputSameDT=on  OutDataTypeStr=Inherit: Same as first input
  Sum : Sum  SaturateOnIntegerOverflow=on  InputSameDT=on  OutDataTypeStr=Inherit: Same as first input
  Sum1 : Sum  Inputs=+-  SaturateOnIntegerOverflow=on  InputSameDT=on  OutDataTypeStr=Inherit: Same as first input
  Sum2 : Sum  Inputs=+-  SaturateOnIntegerOverflow=on  InputSameDT=on  OutDataTypeStr=Inherit: Same as first input
  T : TransportDelay  DelayTime=1/f1  BufferSize=2048
  T1 : TransportDelay  DelayTime=1/f1  BufferSize=2048
  cos(nwt) : Sin  Frequency=2*pi*n*f1  Phase=pi/2  SampleTime=0
  integ1 : Integrator  InitialConditionSource=external
  sin(nwt) : Sin  Frequency=2*pi*n*f1  SampleTime=0
  magnitude : Outport  InitialOutput=0
  angle : Outport  Port=2  InitialOutput=0
  wires:
  Constant/1 -> integ1/2, Integ2/2
  Sum/1 -> Fcn2/1
  Fcn/1 -> Sum/1
  Fcn1/1 -> Sum/2
  Mux/1 -> Fcn3/1
  Fcn3/1 -> angle/1
  sin(nwt)/1 -> Product/1
  cos(nwt)/1 -> Product1/2
  Product/1 -> integ1/1
  Product1/1 -> Integ2/1
  T/1 -> Sum1/2
  T1/1 -> Sum2/2
  integ1/1 -> Sum1/1, T/1
  Integ2/1 -> T1/1, Sum2/1
  Sum2/1 -> Fcn1/1, Mux/2
  Sum1/1 -> Fcn/1, Mux/1
  signal/1 -> Gain1/1
  Gain1/1 -> Product/2, Product1/1
  Fcn2/1 -> magnitude/1

== system power_wind_dfig/Wind Turbine Doubly-Fed Induction Generator (Phasor Type)1/Generator & Converters/Control/wind_dfig_rotor/Power Regulator/Subsystem/Looses ==
  wr : Inport
  idqs : Inport  Port=2
  idq_grid_conv : Inport  Port=3
  idqr : Inport  Port=4
  Constant3 : Constant  Value=R_RL
  Friction Factor : Gain  Gain=F  SaturateOnIntegerOverflow=on  OutDataTypeStr=Inherit: Same as input  ParamDataTypeStr=Inherit: Same as input
  Mean Value : Subsystem  mask(Mean value){Period=1/Fnom}
      mask prompts: Period "Averaging period (s):"
      mask help: This block uses the running window averaging technique to compute the mean value of the input signal over the specified period.
  Product{1..4} (4 alike) : Product  SaturateOnIntegerOverflow=on  InputSameDT=on  OutDataTypeStr=Inherit: Same as first input
  Rr : Constant  Value=Rr
  Rs : Constant  Value=Rs
  Sum2 : Sum  Inputs=+++  SaturateOnIntegerOverflow=on
  Sum5 : Sum  Inputs=|++  SaturateOnIntegerOverflow=on
  id^2+iq^2 : Fcn  Expr=u(1)^2+u(2)^2
  "id^2+iq^2 " : Fcn  Expr=u(1)^2+u(2)^2
  "id^2+iq^2   " : Fcn  Expr=u(1)^2+u(2)^2
  P_looses : Outport
  wires:
  idqr/1 -> "id^2+iq^2 "/1
  idqs/1 -> id^2+iq^2/1
  Mean Value/1(Mean) -> P_looses/1
  Sum5/1 -> Sum2/3
  Product1/1 -> Sum5/2
  Product4/1 -> Sum5/1
  idq_grid_conv/1 -> "id^2+iq^2   "/1
  "id^2+iq^2   "/1 -> Product1/2
  Constant3/1 -> Product1/1
  wr/1 -> Product2/1, Friction Factor/1
  Sum2/1 -> Mean Value/2(Init), Mean Value/1(In)  "Looses"
  Product2/1 -> Sum2/1
  Product3/1 -> Sum2/2
  "id^2+iq^2 "/1 -> Product4/2
  Rr/1 -> Product4/1
  id^2+iq^2/1 -> Product3/2
  Rs/1 -> Product3/1
  Friction Factor/1 -> Product2/2  "T_Friction"

== system power_wind_dfig/Wind Turbine Doubly-Fed Induction Generator (Phasor Type)1/Generator & Converters/Control/wind_dfig_rotor/Power Regulator/Subsystem/Mean Value ==
  note: Mean value
  In : Inport
  Init : Inport  Port=2
  Gain : Gain  Gain=1/Period  SaturateOnIntegerOverflow=on  OutDataTypeStr=Inherit: Same as input  ParamDataTypeStr=Inherit: Same as input
  Step : Step  Time=Period+eps  SampleTime=0
  Sum : Sum  Inputs=+-  SaturateOnIntegerOverflow=on  InputSameDT=on  OutDataTypeStr=Inherit: Same as first input
  Switch : Switch  Threshold=0.5  SaturateOnIntegerOverflow=on
  Transport Delay : TransportDelay  DelayTime=Period
  integrator : Integrator
  Mean : Outport
  wires:
  Transport Delay/1 -> Sum/2
  integrator/1 -> Transport Delay/1, Sum/1
  In/1 -> integrator/1
  Sum/1 -> Gain/1
  Gain/1 -> Switch/1
  Switch/1 -> Mean/1
  Step/1 -> Switch/2
  Init/1 -> Switch/3

== system power_wind_dfig/Wind Turbine Doubly-Fed Induction Generator (Phasor Type)1/Generator & Converters/Control/wind_dfig_rotor/Power Regulator/Subsystem/Slope_B_A ==
  Constant6 : Constant  Value=power_B
  Constant7 : Constant  Value=power_A
  Constant8 : Constant  Value=speed_B
  Constant9 : Constant  Value=speed_A
  Product2 : Product  Inputs=*/  SaturateOnIntegerOverflow=on  OutDataTypeStr=Inherit: Same as first input
  Sum8 : Sum  Inputs=|+-  SaturateOnIntegerOverflow=on
  Sum9 : Sum  Inputs=|+-  SaturateOnIntegerOverflow=on
  Slope : Outport
  wires:
  Constant6/1 -> Sum8/1
  Constant7/1 -> Sum8/2
  Constant8/1 -> Sum9/1
  Constant9/1 -> Sum9/2
  Sum8/1 -> Product2/1
  Sum9/1 -> Product2/2
  Product2/1 -> Slope/1

== system power_wind_dfig/Wind Turbine Doubly-Fed Induction Generator (Phasor Type)1/Generator & Converters/Control/wind_dfig_rotor/Power Regulator/Subsystem/Slope_D_C ==
  Constant2 : Constant  Value=power_D
  Constant3 : Constant  Value=power_C
  Constant4 : Constant  Value=speed_D
  Constant5 : Constant  Value=speed_C
  Product : Product  Inputs=*/  SaturateOnIntegerOverflow=on  OutDataTypeStr=Inherit: Same as first input
  Sum6 : Sum  Inputs=|+-  SaturateOnIntegerOverflow=on
  Sum7 : Sum  Inputs=|+-  SaturateOnIntegerOverflow=on
  Slope : Outport
  wires:
  Constant2/1 -> Sum6/1
  Constant3/1 -> Sum6/2
  Constant4/1 -> Sum7/1
  Constant5/1 -> Sum7/2
  Sum6/1 -> Product/1
  Sum7/1 -> Product/2
  Product/1 -> Slope/1

== system power_wind_dfig/Wind Turbine Doubly-Fed Induction Generator (Phasor Type)1/Generator & Converters/Control/wind_dfig_rotor/Power Regulator/Subsystem/Subsystem2 ==
  In1 : Inport
  Init : Inport  Port=2
  Gain : Gain  Gain=Ki  SaturateOnIntegerOverflow=on  OutDataTypeStr=Inherit: Same as input  ParamDataTypeStr=Inherit: Same as input
  Gain1 : Gain  Gain=Kp  SaturateOnIntegerOverflow=on  OutDataTypeStr=Inherit: Same as input  ParamDataTypeStr=Inherit: Same as input
  Integrator : Integrator  InitialConditionSource=external  InitialCondition=Init  LimitOutput=on  UpperSaturationLimit=Upper_Limit  LowerSaturationLimit=Lower_Limit
  Saturation : Saturate  UpperLimit=Upper_Limit  LowerLimit=Lower_Limit
  Sum7 : Sum  SaturateOnIntegerOverflow=on  InputSameDT=on  OutDataTypeStr=Inherit: Same as first input
  Out1 : Outport
  wires:
  Init/1 -> Integrator/2
  Saturation/1 -> Out1/1
  Sum7/1 -> Saturation/1
  In1/1 -> Gain/1, Gain1/1
  Integrator/1 -> Sum7/2
  Gain1/1 -> Sum7/1
  Gain/1 -> Integrator/1

== system power_wind_dfig/Wind Turbine Doubly-Fed Induction Generator (Phasor Type)1/Generator & Converters/Control/wind_dfig_rotor/Power Regulator/Subsystem /Mean Value ==
  note: Mean value
  In : Inport
  Init : Inport  Port=2
  Gain : Gain  Gain=1/Period  SaturateOnIntegerOverflow=on  OutDataTypeStr=Inherit: Same as input  ParamDataTypeStr=Inherit: Same as input
  Step : Step  Time=Period+eps  SampleTime=0
  Sum : Sum  Inputs=+-  SaturateOnIntegerOverflow=on  InputSameDT=on  OutDataTypeStr=Inherit: Same as first input
  Switch : Switch  Threshold=0.5  SaturateOnIntegerOverflow=on
  Transport Delay : TransportDelay  DelayTime=Period
  integrator : Integrator
  Mean : Outport
  wires:
  Transport Delay/1 -> Sum/2
  integrator/1 -> Transport Delay/1, Sum/1
  In/1 -> integrator/1
  Sum/1 -> Gain/1
  Gain/1 -> Switch/1
  Switch/1 -> Mean/1
  Step/1 -> Switch/2
  Init/1 -> Switch/3

== system power_wind_dfig/Wind Turbine Doubly-Fed Induction Generator (Phasor Type)1/Generator & Converters/Control/wind_dfig_rotor/Power Regulator/Subsystem /Subsystem2 ==
  In1 : Inport
  Init : Inport  Port=2
  Gain : Gain  Gain=Ki  SaturateOnIntegerOverflow=on  OutDataTypeStr=Inherit: Same as input  ParamDataTypeStr=Inherit: Same as input
  Gain1 : Gain  Gain=Kp  SaturateOnIntegerOverflow=on  OutDataTypeStr=Inherit: Same as input  ParamDataTypeStr=Inherit: Same as input
  Integrator : Integrator  InitialConditionSource=external  InitialCondition=Init  LimitOutput=on  UpperSaturationLimit=Upper_Limit  LowerSaturationLimit=Lower_Limit
  Saturation : Saturate  UpperLimit=Upper_Limit  LowerLimit=Lower_Limit
  Sum7 : Sum  SaturateOnIntegerOverflow=on  InputSameDT=on  OutDataTypeStr=Inherit: Same as first input
  Out1 : Outport
  wires:
  Init/1 -> Integrator/2
  Saturation/1 -> Out1/1
  Sum7/1 -> Saturation/1
  In1/1 -> Gain/1, Gain1/1
  Integrator/1 -> Sum7/2
  Gain1/1 -> Sum7/1
  Gain/1 -> Integrator/1

== system power_wind_dfig/Wind Turbine Doubly-Fed Induction Generator (Phasor Type)1/Generator & Converters/Control/wind_dfig_rotor/Power Regulator/Subsystem/Looses/Mean Value ==
  note: Mean value
  In : Inport
  Init : Inport  Port=2
  Gain : Gain  Gain=1/Period  SaturateOnIntegerOverflow=on  OutDataTypeStr=Inherit: Same as input  ParamDataTypeStr=Inherit: Same as input
  Step : Step  Time=Period+eps  SampleTime=0
  Sum : Sum  Inputs=+-  SaturateOnIntegerOverflow=on  InputSameDT=on  OutDataTypeStr=Inherit: Same as first input
  Switch : Switch  Threshold=0.5  SaturateOnIntegerOverflow=on
  Transport Delay : TransportDelay  DelayTime=Period
  integrator : Integrator
  Mean : Outport
  wires:
  Transport Delay/1 -> Sum/2
  integrator/1 -> Transport Delay/1, Sum/1
  In/1 -> integrator/1
  Sum/1 -> Gain/1
  Gain/1 -> Switch/1
  Switch/1 -> Mean/1
  Step/1 -> Switch/2
  Init/1 -> Switch/3
